simulink model "Serial_Logger_Example"  (R2023b)
settings: Solver=ode3  StartTime=0.0  StopTime=inf  RelTol=1e-3  EnableMultiTasking=on
libraries: arduinosensorlib x1, arduinolib x1
settings Model: FPTRunName=Active  ExtModeTrigDuration=2  Creator=Rafael  LastModifiedBy=Rafael
settings SolverCC: AlgebraicLoopSolver=TrustRegion
settings DataIOCC: LimitDataPoints=on  SaveFormat=Array
settings OptimizationCC: ReuseModelBlockBuffer=off  ExpressionDepthLimit=2147483647  LifeSpan=Inf  MaxStackSize=64
settings DebuggingCC: UnderspecifiedInitializationDetection=Classic  MergeDetectMultiDrivingBlocksExec=none  FcnCallInpInsideContextMsg=warning  UnconnectedInputMsg=warning  UnconnectedOutputMsg=warning  UnconnectedLineMsg=warning  AllowSymbolicDim=off  StateNameClashWarn=warning  SFUnexpectedBacktrackingDiag=warning  SFNoUnconditionalDefaultTransitionDiag=warning  SFExecutionAtInitializationDiag=none  ArithmeticOperatorsInVariantConditions=warning
settings HardwareCC: ProdBitPerPointer=32  ProdBitPerSizeT=32  ProdBitPerPtrDiffT=32  ProdLargestAtomicInteger=Long  ProdLargestAtomicFloat=Double  ProdWordSize=32  ProdHWDeviceType=ARM Compatible->ARM Cortex
settings ModelReferenceCC: EnableRefExpFcnMdlSchedulingChecks=on  PropagateSignalLabelsOutOfModel=off
settings SFSimCC: SimUseLocalCustomCode=off  CustomCodeUndefinedFunction=UseInterfaceOnly
settings RTWCC: Description=Embedded Coder  SystemTargetFile=ert.tlc  HardwareBoard=Arduino Due  TemplateMakefile=ert_default_tmf  GenerateReport=on  RTWVerbose=off  RTWUseLocalCustomCode=off  Toolchain=Arduino ARM  BuildConfiguration=Faster Runs  LaunchReport=on
settings CodeAppCC: ForceParamTrailComments=on  OperatorAnnotations=on  StateflowObjectComments=on  MATLABSourceComments=on
settings ERTTargetCC: TargetLangStandard=C99 (ISO)  MultiwordLength=2048  ERTCustomFileBanners=off  SupportContinuousTime=on  SupportNonInlinedSFcns=on  RemoveResetFunc=off  SupportVariableSizeSignals=on  ModelStepFunctionPrototypeControlCompliant=off  ExtModeTransport=3  ExtModeStaticAlloc=on  ExtModeAutomaticAllocSize=off  ExtModeStaticAllocSize=24576  ExtModeMexFile=ext_xcp  ExtModeIntrfLevel=Level2 - Open
settings ConfigComp: CovMetricSettings=dw  CovSaveCumulativeToWorkspaceVar=on  CovSaveSingleToWorkspaceVar=on  CovExternalEMLEnable=off  CovSFcnEnable=off

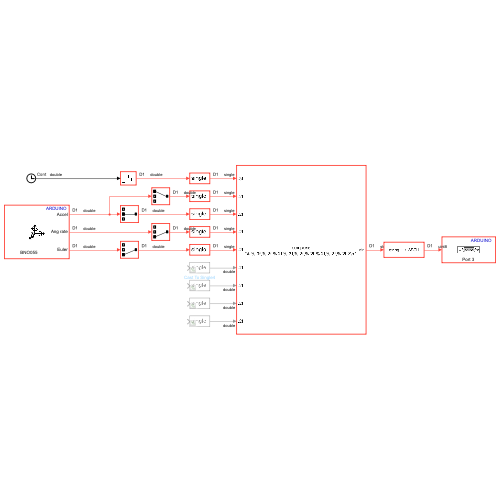
[thumbnail: Simulink's stored preview of the top-level diagram]
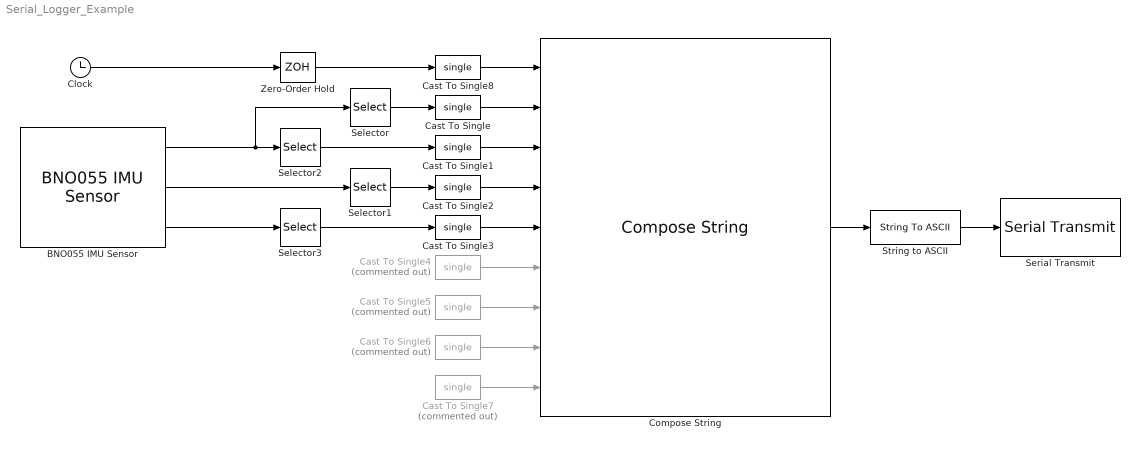
== system Serial_Logger_Example ==
  BNO055 IMU Sensor : arduinosensorlib/BNO055 IMU Sensor  SlaveAddress=0x28  OperationMode=Fusion  Accel=on  AngularRate=on  MagField=off  EulerAngles=on  Quat=off  LinearAccel=off  GravityVector=off  Status=off  Timestamp=off  AccelRange=4G  AccelBW=62.5 Hz  GyroRange=2000 dps  GyroBW=32 Hz  MagODR=10 Hz  spf=1  SampleTime=1/100  blockPlatform=ARDUINO  QueueSizeFactor=1
  Cast To Single{,1..3,8} (5 alike) : DataTypeConversion  OutDataTypeStr=single  SaturateOnIntegerOverflow=off  RndMeth=Floor
  Cast To Single{4..7} (4 alike) : DataTypeConversion  Commented=on  OutDataTypeStr=single  SaturateOnIntegerOverflow=off  RndMeth=Floor
  Clock : Clock
      settings: Decimation=3
  Compose String : ComposeString  Format="\"A,%.3f,%.2f,%.2f,%.2f,%.2f,%.2f,%.2f,%.2f,%.2f,Z\\n\""
  Selector : Selector  InputPortWidth=3  IndexOptions=Index vector (dialog)  Indices=[1]  OutputSizes=1
  Selector1 : Selector  InputPortWidth=3  IndexOptions=Index vector (dialog)  Indices=[3]  OutputSizes=1
  Selector2 : Selector  InputPortWidth=3  IndexOptions=Index vector (dialog)  Indices=[2]  OutputSizes=1
  Selector3 : Selector  InputPortWidth=3  IndexOptions=Index vector (dialog)  Indices=[3]  OutputSizes=1
  Serial Transmit : arduinolib/Serial Transmit  portNumber=3  sendmode=write  sendformat=Decimal  floatprecision=2  blockPlatform=arduino
  String to ASCII : StringToASCII  OutputVectorSize=64
  Zero-Order Hold : ZeroOrderHold  SampleTime=1/100
  wires:
  BNO055 IMU Sensor/1 -> Selector/1, Selector2/1
  BNO055 IMU Sensor/3 -> Selector3/1
  Selector/1 -> Cast To Single/1
  BNO055 IMU Sensor/2 -> Selector1/1
  Selector2/1 -> Cast To Single1/1
  Selector1/1 -> Cast To Single2/1
  Selector3/1 -> Cast To Single3/1
  Cast To Single/1 -> Compose String/2
  Cast To Single1/1 -> Compose String/3
  Cast To Single2/1 -> Compose String/4
  Cast To Single3/1 -> Compose String/5
  Compose String/1 -> String to ASCII/1
  String to ASCII/1 -> Serial Transmit/1
  Clock/1 -> Zero-Order Hold/1
  Cast To Single8/1 -> Compose String/1
  Cast To Single4/1 -> Compose String/6
  Cast To Single5/1 -> Compose String/7
  Cast To Single6/1 -> Compose String/8
  Cast To Single7/1 -> Compose String/9
  Zero-Order Hold/1 -> Cast To Single8/1
